simulink model "ece456PlatRL"  (R2017b)
settings: Solver=ode3  StartTime=0.0  StopTime=inf  RelTol=1e-3
InitFcn:
  | K = [0.4175    0.5498]; %Velocity Control Gains
undefined symbols (not defined in the file or in its folder): DiscIntNeverNeededParam
libraries: legoev3lib x8, simulink x6, simulink_extras x1
CloseFcn:
  | clear K
settings Model: ExtModeTrigDuration=2  Creator=The MathWorks, Inc.  LastModifiedBy=b
settings SolverCC: PositivePriorityOrder=on
settings DataIOCC: LimitDataPoints=on  SaveFormat=Array
settings OptimizationCC: LifeSpan=Inf  MaxStackSize=64
settings DebuggingCC: UnderspecifiedInitializationDetection=Classic  MergeDetectMultiDrivingBlocksExec=none  IntegerOverflowMsg=none  AllowSymbolicDim=off  SFUnexpectedBacktrackingDiag=warning  SFNoUnconditionalDefaultTransitionDiag=warning  SFExecutionAtInitializationDiag=none  IntegerSaturationMsg=none
settings HardwareCC: ProdBitPerPointer=32  ProdBitPerSizeT=32  ProdBitPerPtrDiffT=32  ProdLargestAtomicInteger=Long  ProdWordSize=32  ProdHWDeviceType=ARM Compatible->ARM 9  UseEmbeddedCoderFeatures=off  UseSimulinkCoderFeatures=off
settings ModelReferenceCC: PropagateSignalLabelsOutOfModel=off
settings RTWCC: SystemTargetFile=ert.tlc  HardwareBoard=LEGO MINDSTORMS EV3  TemplateMakefile=ert_default_tmf  GenerateReport=on  RTWVerbose=off  Toolchain=Sourcery G++ Lite v2009q3  BuildConfiguration=Faster Runs  LaunchReport=on
settings CodeAppCC: ForceParamTrailComments=on  OperatorAnnotations=on  StateflowObjectComments=on  MATLABSourceComments=on
settings ERTTargetCC: MultiwordLength=2048  ERTCustomFileBanners=off  SupportContinuousTime=on  SupportNonInlinedSFcns=on  RemoveResetFunc=off  ModelStepFunctionPrototypeControlCompliant=off
settings ConfigComp: CovMetricSettings=dw  CovHtmlReporting=on  CovSaveCumulativeToWorkspaceVar=on  CovSaveSingleToWorkspaceVar=on  CovExternalEMLEnable=off  CovSFcnEnable=off

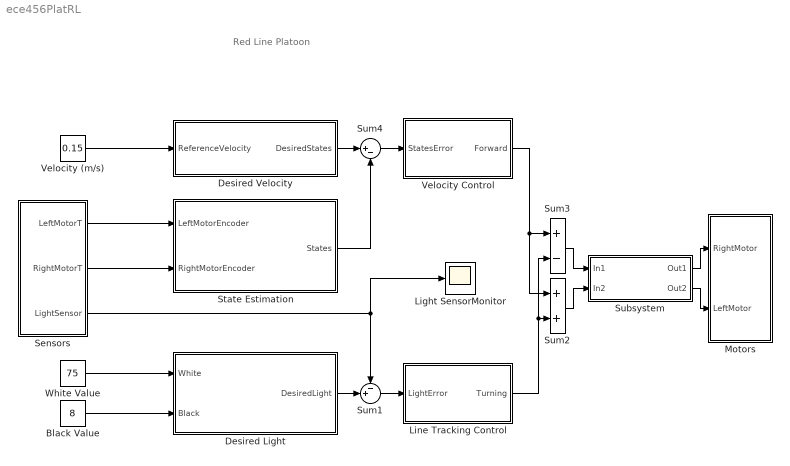
== system ece456PlatRL ==
  note: Red Line Platoon
  Black Value : Constant  Value=8
  Desired Light : Subsystem
  Desired Velocity : Subsystem
  Light SensorMonitor : Scope
  "Line Tracking Control " : Subsystem
  Motors : Subsystem
  Sensors : Subsystem
  State Estimation : Subsystem
  Subsystem : Subsystem
  Sum1 : Sum  Inputs=-+|
  Sum2 : Sum
  Sum3 : Sum  Inputs=+-
  Sum4 : Sum  Inputs=|+-
  Velocity (m/s) : Constant  Value=0.15
  Velocity Control : Subsystem
  White Value : Constant  Value=75
  wires:
  Desired Light/1(DesiredLight) -> Sum1/2
  "Line Tracking Control "/1(Turning) -> Sum2/2, Sum3/2
  Sum1/1 -> "Line Tracking Control "/1(LightError)
  State Estimation/1(States) -> Sum4/2
  Velocity (m/s)/1 -> Desired Velocity/1(ReferenceVelocity)
  Desired Velocity/1(DesiredStates) -> Sum4/1
  Velocity Control/1(Forward) -> Sum2/1, Sum3/1
  Sum4/1 -> Velocity Control/1(StatesError)
  White Value/1 -> Desired Light/1(White)
  Black Value/1 -> Desired Light/2(Black)
  Sensors/3(LightSensor) -> Sum1/1, Light SensorMonitor/1
  Sensors/1(LeftMotorT) -> State Estimation/1(LeftMotorEncoder)
  Sensors/2(RightMotorT) -> State Estimation/2(RightMotorEncoder)
  Sum3/1 -> Subsystem/1(In1)
  Subsystem/1(Out1) -> Motors/1(RightMotor)
  Sum2/1 -> Subsystem/2(In2)
  Subsystem/2(Out2) -> Motors/2(LeftMotor)

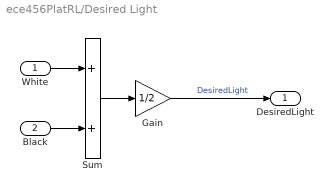
== system ece456PlatRL/Desired Light ==
  White : Inport
  Black : Inport  Port=2
  Gain : Gain  Gain=1/2
  Sum : Sum
  DesiredLight : Outport
  wires:
  Sum/1 -> Gain/1
  White/1 -> Sum/1
  Black/1 -> Sum/2
  Gain/1 -> DesiredLight/1  "DesiredLight"

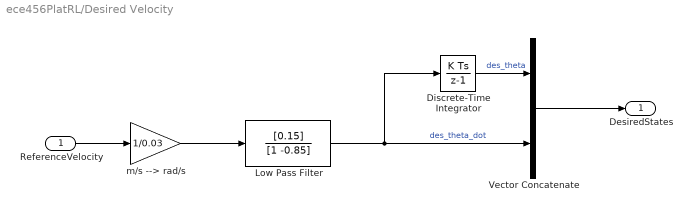
== system ece456PlatRL/Desired Velocity ==
  ReferenceVelocity : Inport
  Discrete-Time Integrator : DiscreteIntegrator  SampleTime=-1  ICPrevOutput=DiscIntNeverNeededParam  ICPrevScaledInput=DiscIntNeverNeededParam
  Low Pass Filter : DiscreteFilter  Numerator=[0.15]  Denominator=[1 -0.85]
  Vector Concatenate : Concatenate
  m/s --> rad/s : Gain  Gain=1/0.03
  DesiredStates : Outport
  wires:
  Vector Concatenate/1 -> DesiredStates/1
  ReferenceVelocity/1 -> m/s --> rad/s/1
  m/s --> rad/s/1 -> Low Pass Filter/1
  Discrete-Time Integrator/1 -> Vector Concatenate/1  "des_theta"
  Low Pass Filter/1 -> Discrete-Time Integrator/1, Vector Concatenate/2  "des_theta_dot"

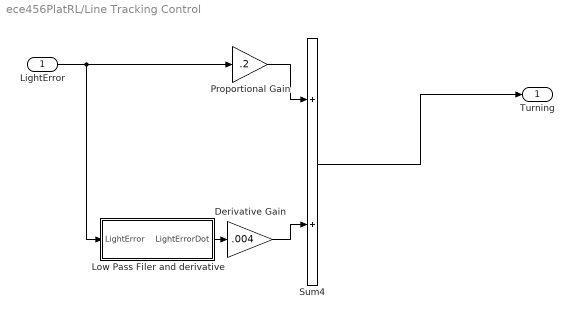
== system ece456PlatRL/Line Tracking Control  ==
  LightError : Inport
  Derivative Gain : Gain  Gain=.004
  Low Pass Filer and derivative : Subsystem
  Proportional Gain : Gain  Gain=.2
  Sum4 : Sum
  Turning : Outport
  wires:
  LightError/1 -> Low Pass Filer and derivative/1(LightError), Proportional Gain/1
  Low Pass Filer and derivative/1(LightErrorDot) -> Derivative Gain/1
  Derivative Gain/1 -> Sum4/2
  Proportional Gain/1 -> Sum4/1
  Sum4/1 -> Turning/1

== system ece456PlatRL/Motors ==
  RightMotor : Inport
  LeftMotor : Inport  Port=2
  " Left Motor" : legoev3lib/Motor  sportNumber=B  sstopAction=Brake
  Right Motor : legoev3lib/Motor  sportNumber=C  sstopAction=Brake
  wires:
  RightMotor/1 -> Right Motor/1
  LeftMotor/1 -> " Left Motor"/1

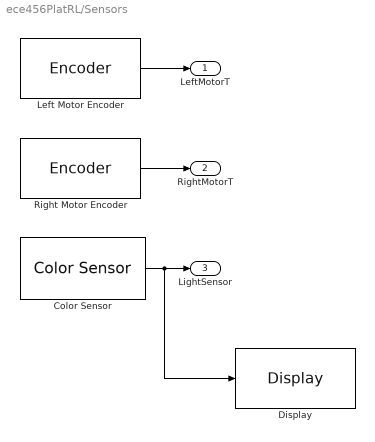
== system ece456PlatRL/Sensors ==
  Color Sensor : legoev3lib/Color Sensor  portNumber=4  mode=Reflected light intensity  sampleTime=0.004
      settings: SourceProductName=Simulink Support Package for LEGO MINDSTORMS EV3 Hardware  SourceProductBaseCode=LEGOEV3
  Display : legoev3lib/Display  slcdStr=light  slcdLine=1  slcdFormat=Decimal
      settings: SourceProductName=Simulink Support Package for LEGO MINDSTORMS EV3 Hardware  SourceProductBaseCode=LEGOEV3
  Left Motor Encoder : legoev3lib/Encoder  portNumber=B  opMode=No reset  sampleTime=0.004
      settings: SourceProductName=Simulink Support Package for LEGO MINDSTORMS EV3 Hardware  SourceProductBaseCode=LEGOEV3
  Right Motor Encoder : legoev3lib/Encoder  portNumber=C  opMode=No reset  sampleTime=0.004
      settings: SourceProductName=Simulink Support Package for LEGO MINDSTORMS EV3 Hardware  SourceProductBaseCode=LEGOEV3
  LeftMotorT : Outport
  RightMotorT : Outport  Port=2
  LightSensor : Outport  Port=3
  wires:
  Left Motor Encoder/1 -> LeftMotorT/1
  Right Motor Encoder/1 -> RightMotorT/1
  Color Sensor/1 -> Display/1, LightSensor/1

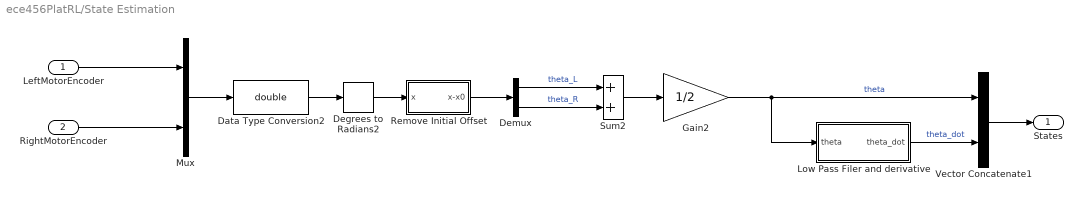
== system ece456PlatRL/State Estimation ==
  LeftMotorEncoder : Inport
  RightMotorEncoder : Inport  Port=2
  Data Type Conversion2 : DataTypeConversion  OutDataTypeStr=double
  Degrees to Radians2 : simulink_extras/Transformations/Degrees to Radians
  Demux : Demux  Outputs=2
  Gain2 : Gain  Gain=1/2
  Low Pass Filer and derivative : Subsystem
  Mux : Mux  Inputs=2
  Remove Initial Offset : Subsystem
  Sum2 : Sum
  Vector Concatenate1 : Concatenate
  States : Outport
  wires:
  Remove Initial Offset/1(x-x0) -> Demux/1
  LeftMotorEncoder/1 -> Mux/1
  RightMotorEncoder/1 -> Mux/2
  Demux/1 -> Sum2/1  "theta_L"
  Demux/2 -> Sum2/2  "theta_R"
  Vector Concatenate1/1 -> States/1
  Gain2/1 -> Low Pass Filer and derivative/1(theta), Vector Concatenate1/1  "theta"
  Sum2/1 -> Gain2/1
  Data Type Conversion2/1 -> Degrees to Radians2/1
  Degrees to Radians2/1 -> Remove Initial Offset/1(x)
  Mux/1 -> Data Type Conversion2/1
  Low Pass Filer and derivative/1(theta_dot) -> Vector Concatenate1/2  "theta_dot"

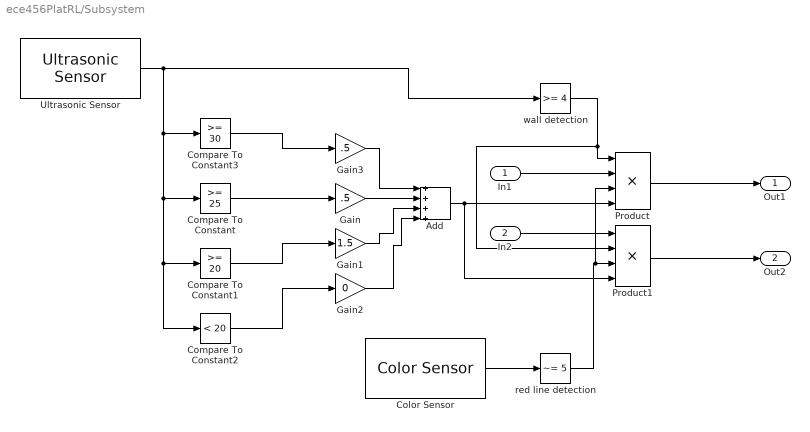
== system ece456PlatRL/Subsystem ==
  In1 : Inport
  In2 : Inport  Port=2
  Add : Sum  Inputs=++++
  Color Sensor : legoev3lib/Color Sensor  portNumber=1  mode=Color  sampleTime=0.1
      settings: SourceProductName=Simulink Support Package for LEGO MINDSTORMS EV3 Hardware  SourceProductBaseCode=LEGOEV3
  Compare To Constant : simulink/Logic and Bit Operations/Compare To Constant  relop=>=  const=25  OutDataTypeStr=boolean
  Compare To Constant1 : simulink/Logic and Bit Operations/Compare To Constant  relop=>=  const=20  OutDataTypeStr=boolean
  Compare To Constant2 : simulink/Logic and Bit Operations/Compare To Constant  relop=<  const=20  OutDataTypeStr=boolean
  Compare To Constant3 : simulink/Logic and Bit Operations/Compare To Constant  relop=>=  const=30  OutDataTypeStr=boolean
  Gain : Gain  Gain=.5
  Gain1 : Gain  Gain=1.5
  Gain2 : Gain  Gain=0
  Gain3 : Gain  Gain=.5
  Product : Product  Inputs=4
  Product1 : Product  Inputs=4
  Ultrasonic Sensor : legoev3lib/Ultrasonic Sensor  PortNumber=3  sampleTime=0.004
      settings: SourceProductName=Simulink Support Package for LEGO MINDSTORMS EV3 Hardware  SourceProductBaseCode=LEGOEV3
  red line detection : simulink/Logic and Bit Operations/Compare To Constant  relop=~=  const=5  OutDataTypeStr=boolean
  wall detection : simulink/Logic and Bit Operations/Compare To Constant  relop=>=  const=4  OutDataTypeStr=boolean
  Out1 : Outport
  Out2 : Outport  Port=2
  wires:
  In1/1 -> Product/2
  wall detection/1 -> Product1/2, Product/1
  Ultrasonic Sensor/1 -> Compare To Constant3/1, Compare To Constant2/1, Compare To Constant1/1, Compare To Constant/1, wall detection/1
  Product/1 -> Out1/1
  In2/1 -> Product1/1
  Product1/1 -> Out2/1
  Color Sensor/1 -> red line detection/1
  red line detection/1 -> Product/3, Product1/3
  Compare To Constant2/1 -> Gain2/1
  Compare To Constant1/1 -> Gain1/1
  Compare To Constant/1 -> Gain/1
  Add/1 -> Product1/4, Product/4
  Gain2/1 -> Add/4
  Gain1/1 -> Add/3
  Gain/1 -> Add/2
  Compare To Constant3/1 -> Gain3/1
  Gain3/1 -> Add/1

== system ece456PlatRL/Velocity Control ==
  StatesError : Inport
  " State Feedback [Ki Kp] %Change these values in the model's InitFcn callback" : Gain  Gain=K  Multiplication=Matrix(K*u)
  Convert Volt to PWM : Subsystem
  Forward : Outport
  wires:
  StatesError/1 -> " State Feedback [Ki Kp] %Change these values in the model's InitFcn callback"/1
  " State Feedback [Ki Kp] %Change these values in the model's InitFcn callback"/1 -> Convert Volt to PWM/1(Volt Cmd)
  Convert Volt to PWM/1(PWM) -> Forward/1

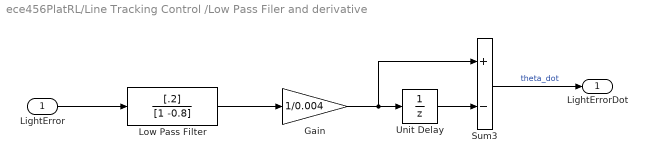
== system ece456PlatRL/Line Tracking Control /Low Pass Filer and derivative ==
  LightError : Inport
  Gain : Gain  Gain=1/0.004
  Low Pass Filter : DiscreteFilter  Numerator=[.2]  Denominator=[1 -0.8]
  Sum3 : Sum  Inputs=+-
  Unit Delay : UnitDelay  SampleTime=-1
  LightErrorDot : Outport
  wires:
  Unit Delay/1 -> Sum3/2
  Gain/1 -> Unit Delay/1, Sum3/1
  Sum3/1 -> LightErrorDot/1  "theta_dot"
  Low Pass Filter/1 -> Gain/1
  LightError/1 -> Low Pass Filter/1

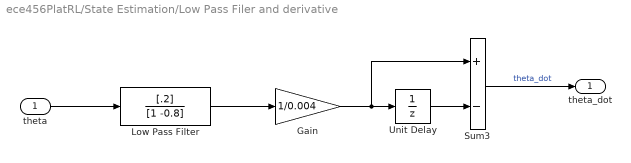
== system ece456PlatRL/State Estimation/Low Pass Filer and derivative ==
  theta : Inport
  Gain : Gain  Gain=1/0.004
  Low Pass Filter : DiscreteFilter  Numerator=[.2]  Denominator=[1 -0.8]
  Sum3 : Sum  Inputs=+-
  Unit Delay : UnitDelay  SampleTime=-1
  theta_dot : Outport
  wires:
  Unit Delay/1 -> Sum3/2
  Gain/1 -> Unit Delay/1, Sum3/1
  Sum3/1 -> theta_dot/1  "theta_dot"
  Low Pass Filter/1 -> Gain/1
  theta/1 -> Low Pass Filter/1

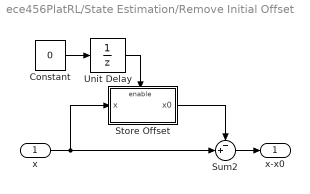
== system ece456PlatRL/State Estimation/Remove Initial Offset ==
  x : Inport
  Constant : Constant  Value=0  OutDataTypeStr=boolean
  Store Offset : Subsystem  TreatAsAtomicUnit=on
  Sum2 : Sum  Inputs=-+|
  Unit Delay : UnitDelay  InitialCondition=1  SampleTime=-1
  x-x0 : Outport
  wires:
  Sum2/1 -> x-x0/1
  Unit Delay/1 -> Store Offset/Enable
  Constant/1 -> Unit Delay/1
  Store Offset/1(x0) -> Sum2/1
  x/1 -> Store Offset/1(x), Sum2/2

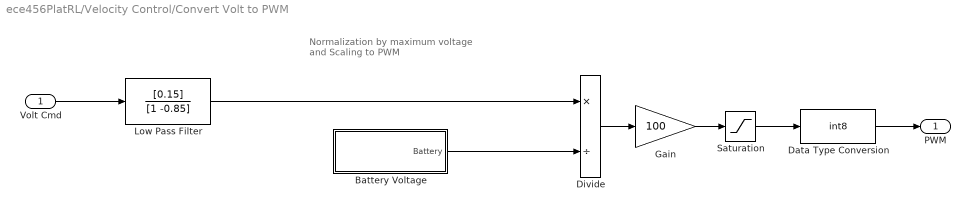
== system ece456PlatRL/Velocity Control/Convert Volt to PWM ==
  note: Normalization by maximum voltage
      | and
      | Scaling to PWM
  Volt Cmd : Inport
  Battery Voltage : Subsystem
  Data Type Conversion : DataTypeConversion  OutDataTypeStr=int8
  Divide : Product  Inputs=*/
  Gain : Gain  Gain=100
  Low Pass Filter : DiscreteFilter  Numerator=[0.15]  Denominator=[1 -0.85]
  Saturation : Saturate  UpperLimit=100  LowerLimit=-100
  PWM : Outport
  wires:
  Data Type Conversion/1 -> PWM/1
  Saturation/1 -> Data Type Conversion/1
  Volt Cmd/1 -> Low Pass Filter/1
  Gain/1 -> Saturation/1
  Divide/1 -> Gain/1
  Low Pass Filter/1 -> Divide/1
  Battery Voltage/1(Battery) -> Divide/2

== system ece456PlatRL/State Estimation/Remove Initial Offset/Store Offset ==
  x : Inport
  Enable : EnablePort
  x0 : Outport  InitialOutput=0
  wires:
  x/1 -> x0/1

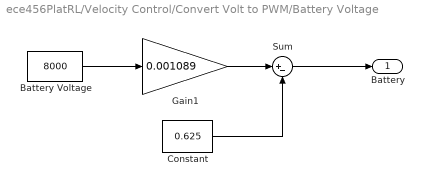
== system ece456PlatRL/Velocity Control/Convert Volt to PWM/Battery Voltage ==
  Battery Voltage : Constant  Value=8000
  Constant : Constant  Value=0.625
  Gain1 : Gain  Gain=0.001089
  Sum : Sum  Inputs=|+-
  Battery : Outport
  wires:
  Sum/1 -> Battery/1
  Battery Voltage/1 -> Gain1/1
  Constant/1 -> Sum/2
  Gain1/1 -> Sum/1
